simulink model "NewAuto_V1"  (R2021a)
settings: Solver=FixedStepAuto  StartTime=0.0  StopTime=inf  RelTol=1e-3
libraries: vexarmcortexlib x28, vexcommonlib x8
settings Model: ExtModeTrigDuration=25  Creator=nicoa  LastModifiedBy=Mihai Nicoara
settings SolverCC: AlgebraicLoopSolver=TrustRegion
settings OptimizationCC: EnhancedBackFolding=on  PassReuseOutputArgsAs=Individual arguments  ZeroExternalMemoryAtStartup=off  ZeroInternalMemoryAtStartup=off  MaxStackSize=64  OptimizeBlockOrder=speed  DifferentSizesBufferReuse=on  OptimizationCustomize=off  EfficientTunableParamExpr=on
settings DebuggingCC: ParameterTunabilityLossMsg=error  SFMachineParentedDataDiag=warning
settings HardwareCC: ProdBitPerPointer=32  ProdBitPerSizeT=32  ProdBitPerPtrDiffT=32  ProdLargestAtomicInteger=Long  ProdLargestAtomicFloat=Double  ProdWordSize=32  ProdHWDeviceType=ARM Compatible->ARM Cortex
settings SFSimCC: MATLABDynamicMemAlloc=off
settings RTWCC: SystemTargetFile=ert.tlc  HardwareBoard=ARM Cortex-based VEX Microcontroller  TLCOptions="-aInlineSetEventsForThisBaseRateFcn=TLC_FALSE -aSuppressMultiTaskScheduler=TLC_FALSE  -aRateBasedStepFcn=0"  TemplateMakefile=ert_default_tmf  GenerateReport=on  Toolchain=GNU Tools for VEX ARM Cortex  IncludeHyperlinkInReport=on  LaunchReport=on  GenerateTraceInfo=on  GenerateTraceReport=on  GenerateTraceReportSl=on  GenerateTraceReportSf=on  GenerateTraceReportEml=on
settings CodeAppCC: ForceParamTrailComments=on  IgnoreCustomStorageClasses=off  OperatorAnnotations=on  SimulinkDataObjDesc=on  SFDataObjDesc=on  InsertBlockDesc=on

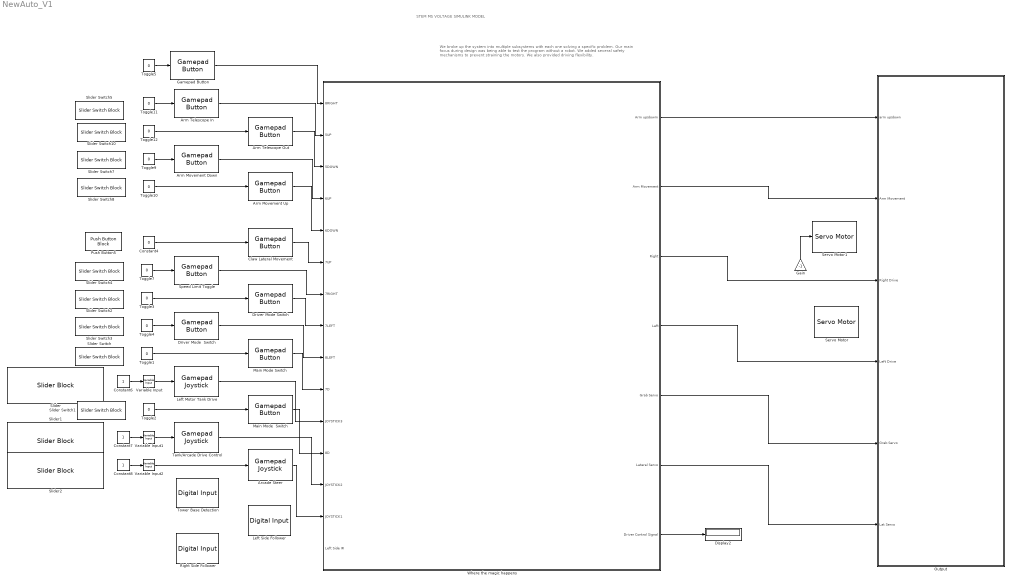
== system NewAuto_V1 ==
  note: We broke up the system into multiple subsystems with each one solving a specific problem. Our main focus during
      | design was being able to test the program without a robot. We added several safety mechanisms to prevent straining
      |  the motors. We also provided driving flexibility.
  note: STEM MS VOLTAGE SIMULINK MODEL
  "Arcade Steer " : vexarmcortexlib/Gamepad/Gamepad Joystick  joystick=1  chan=1  SimulationIn=on  SampleTime=0.02
      settings: SourceProductBaseCode=EC_VEX_MICRO
  Arm Movement Down : vexarmcortexlib/Gamepad/Gamepad Button  joystick=1  chan=6  button56=Down  button78=Down  SimulationIn=on  SampleTime=0.02
      settings: SourceProductBaseCode=EC_VEX_MICRO
  Arm Movement Up : vexarmcortexlib/Gamepad/Gamepad Button  joystick=1  chan=6  button56=Up  button78=Down  SimulationIn=on  SampleTime=0.02
      settings: SourceProductBaseCode=EC_VEX_MICRO
  Arm Telescope In : vexarmcortexlib/Gamepad/Gamepad Button  joystick=1  chan=5  button56=Down  button78=Down  SimulationIn=on  SampleTime=0.02
      settings: SourceProductBaseCode=EC_VEX_MICRO
  Arm Telescope Out : vexarmcortexlib/Gamepad/Gamepad Button  joystick=1  chan=5  button56=Up  button78=Down  SimulationIn=on  SampleTime=0.02
      settings: SourceProductBaseCode=EC_VEX_MICRO
  Claw Lateral Movement : vexarmcortexlib/Gamepad/Gamepad Button  joystick=1  chan=7  button56=Up  button78=Up  SimulationIn=on  SampleTime=0.02
      settings: SourceProductBaseCode=EC_VEX_MICRO
  Constant4 : Constant  Value=0
  Constant6 : Constant
  Constant7 : Constant
  Constant8 : Constant
  Display2 : Display
  Driver Mode  Switch : vexarmcortexlib/Gamepad/Gamepad Button  joystick=1  chan=8  button56=Up  button78=Left  SimulationIn=on  SampleTime=0.02
      settings: SourceProductBaseCode=EC_VEX_MICRO
  Driver Mode Switch : vexarmcortexlib/Gamepad/Gamepad Button  joystick=1  chan=7  button56=Up  button78=Left  SimulationIn=on  SampleTime=0.02
      settings: SourceProductBaseCode=EC_VEX_MICRO
  Gain : Gain  Gain=-1
  Gamepad Button : vexarmcortexlib/Gamepad/Gamepad Button  joystick=1  chan=8  button56=Up  button78=Right  SimulationIn=on  SampleTime=0.02
      settings: SourceProductBaseCode=EC_VEX_MICRO
  Left Motor Tank Drive : vexarmcortexlib/Gamepad/Gamepad Joystick  joystick=1  chan=3  SimulationIn=on  SampleTime=0.02
      settings: SourceProductBaseCode=EC_VEX_MICRO
  Left Side Follower : vexarmcortexlib/Sensors/Digital Input  inChan=1  SimulationIn=off  SampleTime=0.002
      settings: SourceProductBaseCode=EC_VEX_MICRO
  Main Mode  Switch : vexarmcortexlib/Gamepad/Gamepad Button  joystick=1  chan=8  button56=Up  button78=Down  SimulationIn=on  SampleTime=0.02
      settings: SourceProductBaseCode=EC_VEX_MICRO
  Main Mode Switch : vexarmcortexlib/Gamepad/Gamepad Button  joystick=1  chan=7  button56=Up  button78=Down  SimulationIn=on  SampleTime=0.02
      settings: SourceProductBaseCode=EC_VEX_MICRO
  Output : Subsystem
  Push Button5 : PushButtonBlock
  Right Side Follower : vexarmcortexlib/Sensors/Digital Input  inChan=6  SimulationIn=off  SampleTime=0.002
      settings: SourceProductBaseCode=EC_VEX_MICRO
  Servo Motor : vexarmcortexlib/Actuators/Servo Motor  motor=5  scaleFactor=60/127  SimulationOut=off
      settings: SourceProductBaseCode=EC_VEX_MICRO
  Servo Motor1 : vexarmcortexlib/Actuators/Servo Motor  motor=6  scaleFactor=60/127  SimulationOut=off
      settings: SourceProductBaseCode=EC_VEX_MICRO
  Slider : SliderBlock  LabelPosition=Hide  ScaleMin=-127  ScaleMax=127
  Slider Switch{,1..5,7..8,10} (9 alike) : SliderSwitchBlock  LabelPosition=Hide
      settings: Values={{'Off', 'On'}, [0 1]}
  Slider1 : SliderBlock  LabelPosition=Hide  ScaleMin=-127  ScaleMax=127
  Slider2 : SliderBlock  LabelPosition=Hide  ScaleMin=-127  ScaleMax=127
  Speed Limit Toggle : vexarmcortexlib/Gamepad/Gamepad Button  joystick=1  chan=7  button56=Up  button78=Right  SimulationIn=on  SampleTime=0.02
      settings: SourceProductBaseCode=EC_VEX_MICRO
  Tank/Arcade Drive Control : vexarmcortexlib/Gamepad/Gamepad Joystick  joystick=1  chan=2  SimulationIn=on  SampleTime=0.02
      settings: SourceProductBaseCode=EC_VEX_MICRO
  Toggle{1..5,7,9..12} (10 alike) : Constant  Value=0
      settings: OpenFcn=|
      | if strcmp('0',get_param(gcb, 'Value'))                        set_param(gcb, 'Value', '1');
      | else
      |             set_param(gcb, 'Value', '0');
      | end
  Tower Base Detection : vexarmcortexlib/Sensors/Digital Input  inChan=11  SimulationIn=off  SampleTime=0.002
      settings: SourceProductBaseCode=EC_VEX_MICRO
  Variable Input : vexarmcortexlib/Utilities/Variable Input  low=-127  gain=-29.69085144927537  high=127
      settings: SourceProductBaseCode=EC_VEX_MICRO
  Variable Input1 : vexarmcortexlib/Utilities/Variable Input  low=-127  gain=0  high=127
      settings: SourceProductBaseCode=EC_VEX_MICRO
  Variable Input2 : vexarmcortexlib/Utilities/Variable Input  low=-127  gain=0  high=127
      settings: SourceProductBaseCode=EC_VEX_MICRO
  Where the magic happens : Subsystem
  wires:
  Main Mode  Switch/1 -> Where the magic happens/12(8D)
  Main Mode Switch/1 -> Where the magic happens/10(7D)
  Driver Mode  Switch/1 -> Where the magic happens/9(8LEFT)
  Driver Mode Switch/1 -> Where the magic happens/8(7LEFT)
  Speed Limit Toggle/1 -> Where the magic happens/7(7RIGHT)
  Tank/Arcade Drive Control/1 -> Where the magic happens/13(JOYSTICK2)
  Left Motor Tank Drive/1 -> Where the magic happens/11(JOYSTICK3)
  "Arcade Steer "/1 -> Where the magic happens/14(JOYSTICK1)
  Claw Lateral Movement/1 -> Where the magic happens/6(7UP)
  Arm Movement Up/1 -> Where the magic happens/5(6DOWN)
  Arm Movement Down/1 -> Where the magic happens/4(6UP)
  Arm Telescope Out/1 -> Where the magic happens/3(5DOWN)
  Arm Telescope In/1 -> Where the magic happens/2(5UP)
  Toggle11/1 -> Arm Telescope In/1
  Toggle12/1 -> Arm Telescope Out/1
  Toggle9/1 -> Arm Movement Down/1
  Toggle10/1 -> Arm Movement Up/1
  Constant4/1 -> Claw Lateral Movement/1
  Toggle7/1 -> Speed Limit Toggle/1
  Toggle4/1 -> Driver Mode  Switch/1
  Toggle1/1 -> Main Mode Switch/1
  Constant6/1 -> Variable Input/1
  Variable Input/1 -> Left Motor Tank Drive/1
  Variable Input1/1 -> Tank/Arcade Drive Control/1
  Constant7/1 -> Variable Input1/1
  Variable Input2/1 -> "Arcade Steer "/1
  Constant8/1 -> Variable Input2/1
  Toggle2/1 -> Main Mode  Switch/1
  Toggle3/1 -> Driver Mode Switch/1
  Where the magic happens/7(Driver Control Signal) -> Display2/1
  Where the magic happens/6(Lateral Servo) -> Output/6(Lat Servo)
  Where the magic happens/5(Grab Servo) -> Output/5(Grab Servo)
  Where the magic happens/1(Arm up/dowm) -> Output/1(arm up/down)
  Where the magic happens/2(Arm Movement) -> Output/2(Arm Movement)
  Toggle5/1 -> Gamepad Button/1
  Gamepad Button/1 -> Where the magic happens/1(8RIGHT)
  Where the magic happens/3(Right) -> Output/3(Right Drive)
  Where the magic happens/4(Left) -> Output/4(Left Drive)
  ? -> Servo Motor/1, Gain/1
  Gain/1 -> Servo Motor1/1

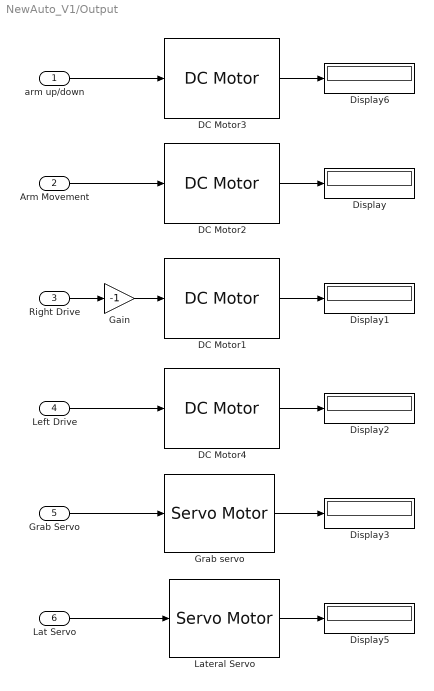
== system NewAuto_V1/Output ==
  arm up/down : Inport
  Arm Movement : Inport  Port=2
  Right Drive : Inport  Port=3
  Left Drive : Inport  Port=4
  Grab Servo : Inport  Port=5
  Lat Servo : Inport  Port=6
  DC Motor1 : vexarmcortexlib/Actuators/DC Motor  motor=2  scaleFactor=1/13.5  SimulationOut=on
      settings: SourceProductBaseCode=EC_VEX_MICRO
  DC Motor2 : vexarmcortexlib/Actuators/DC Motor  motor=4  scaleFactor=1/13.5  SimulationOut=on
      settings: SourceProductBaseCode=EC_VEX_MICRO
  DC Motor3 : vexarmcortexlib/Actuators/DC Motor  motor=7  scaleFactor=1/13.5  SimulationOut=on
      settings: SourceProductBaseCode=EC_VEX_MICRO
  DC Motor4 : vexarmcortexlib/Actuators/DC Motor  motor=9  scaleFactor=1/13.5  SimulationOut=on
      settings: SourceProductBaseCode=EC_VEX_MICRO
  Display{,1..3,5..6} (6 alike) : Display
  Gain : Gain  Gain=-1
  Grab servo : vexarmcortexlib/Actuators/Servo Motor  motor=3  scaleFactor=60/127  SimulationOut=on
      settings: SourceProductBaseCode=EC_VEX_MICRO
  Lateral Servo : vexarmcortexlib/Actuators/Servo Motor  motor=8  scaleFactor=60/127  SimulationOut=on
      settings: SourceProductBaseCode=EC_VEX_MICRO
  wires:
  Grab servo/1 -> Display3/1
  Arm Movement/1 -> DC Motor2/1
  Grab Servo/1 -> Grab servo/1
  DC Motor2/1 -> Display/1
  DC Motor3/1 -> Display6/1
  DC Motor4/1 -> Display2/1
  DC Motor1/1 -> Display1/1
  Lateral Servo/1 -> Display5/1
  arm up/down/1 -> DC Motor3/1
  Lat Servo/1 -> Lateral Servo/1
  Right Drive/1 -> Gain/1
  Left Drive/1 -> DC Motor4/1
  Gain/1 -> DC Motor1/1

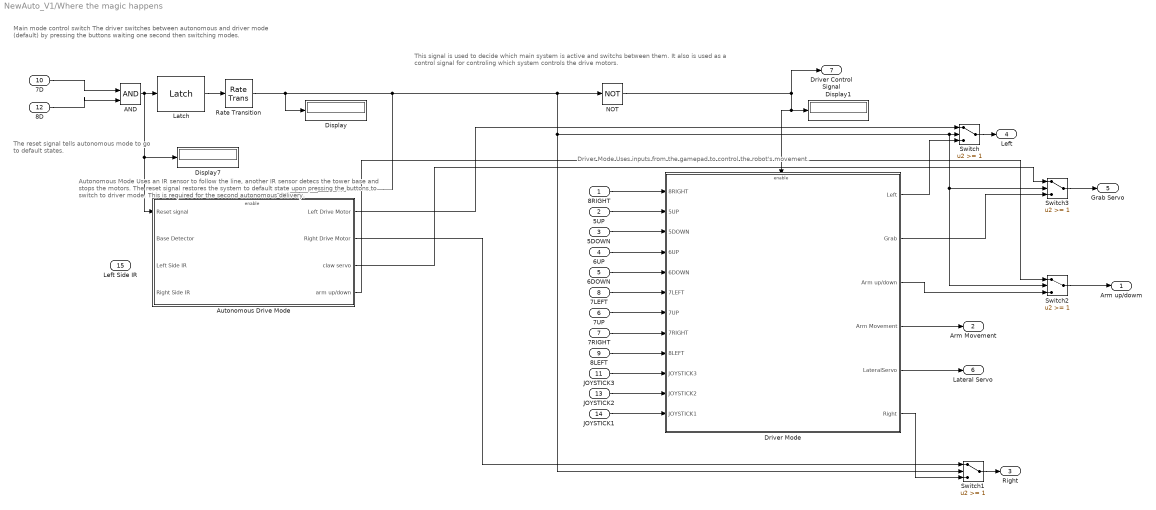
== system NewAuto_V1/Where the magic happens ==
  note: Driver Mode
      | Uses inputs from the gamepad to control the robot's movement.
  note: This signal is used to decide which main system is active and switchs between them.
      | It also is used as a control signal for controling which system controls the drive motors.
  note: The reset signal tells autonomous
      | mode to go to default states.
  note: Autonomous Mode
      | 	Uses an IR sensor to follow the line, another IR sensor detecs the
      | 	tower base and stops the motors. The reset signal restores the system
      | 	to default state upon pressing the buttons to switch to driver mode. This
      | 	is required for the second autonomous delivery.
  note: Main mode control switch
      | The driver switches between autonomous and driver mode (default) by
      | pressing the buttons waiting one second then switching modes.
  8RIGHT : Inport
  5UP : Inport  Port=2
  5DOWN : Inport  Port=3
  6UP : Inport  Port=4
  6DOWN : Inport  Port=5
  7UP : Inport  Port=6
  7RIGHT : Inport  Port=7
  7LEFT : Inport  Port=8
  8LEFT : Inport  Port=9
  7D : Inport  Port=10
  JOYSTICK3 : Inport  Port=11
  8D : Inport  Port=12
  JOYSTICK2 : Inport  Port=13
  JOYSTICK1 : Inport  Port=14
  Left Side IR : Inport  Port=15
  "AND " : Logic  IconShape=distinctive  AllPortsSameDT=off  OutDataTypeStr=boolean
  Autonomous Drive Mode : Subsystem
  Display : Display
  Display1 : Display
  Display7 : Display
  Driver Mode : Subsystem  TreatAsAtomicUnit=on
  Latch : vexcommonlib/Latch  output0=off  BlockPlatform=vexarmcortex
      settings: SourceProductBaseCode=EC_VEX_MICRO,VEXV5
  NOT : Logic  Operator=NOT  IconShape=distinctive  AllPortsSameDT=off  OutDataTypeStr=boolean
  Rate Transition : RateTransition
  Switch{,1..3} (4 alike) : Switch  Threshold=1
  Arm up/dowm : Outport
  Arm Movement : Outport  Port=2
  Right : Outport  Port=3
  Left : Outport  Port=4
  Grab Servo : Outport  Port=5
  Lateral Servo : Outport  Port=6
  Driver Control Signal : Outport  Port=7
  wires:
  7D/1 -> "AND "/1
  "AND "/1 -> Latch/1, Display7/1, Autonomous Drive Mode/1(Reset signal)
  8D/1 -> "AND "/2
  Rate Transition/1 -> Display/1, Autonomous Drive Mode/Enable, NOT/1, Switch1/2, Switch3/2, Switch2/2, Switch/2
  NOT/1 -> Display1/1, Driver Mode/Enable, Driver Control Signal/1
  Autonomous Drive Mode/1(Left Drive Motor) -> Switch/1
  Switch/1 -> Left/1
  Autonomous Drive Mode/2(Right Drive Motor) -> Switch1/1
  Switch1/1 -> Right/1
  7RIGHT/1 -> Driver Mode/8(7RIGHT)
  JOYSTICK3/1 -> Driver Mode/10(JOYSTICK3)
  JOYSTICK2/1 -> Driver Mode/11(JOYSTICK2)
  JOYSTICK1/1 -> Driver Mode/12(JOYSTICK1)
  7UP/1 -> Driver Mode/7(7UP)
  Driver Mode/4(Arm Movement) -> Arm Movement/1
  Driver Mode/1(Left) -> Switch/3
  5DOWN/1 -> Driver Mode/3(5DOWN)
  5UP/1 -> Driver Mode/2(5UP)
  6UP/1 -> Driver Mode/4(6UP)
  6DOWN/1 -> Driver Mode/5(6DOWN)
  7LEFT/1 -> Driver Mode/6(7LEFT)
  8LEFT/1 -> Driver Mode/9(8LEFT)
  Latch/1 -> Rate Transition/1
  Driver Mode/6(Right) -> Switch1/3
  Driver Mode/5(LateralServo) -> Lateral Servo/1
  8RIGHT/1 -> Driver Mode/1(8RIGHT)
  Switch2/1 -> Arm up/dowm/1
  Autonomous Drive Mode/4(arm up/down) -> Switch2/1
  Driver Mode/3(Arm up/down) -> Switch2/3
  Switch3/1 -> Grab Servo/1
  Autonomous Drive Mode/3(claw servo) -> Switch3/1
  Driver Mode/2(Grab) -> Switch3/3

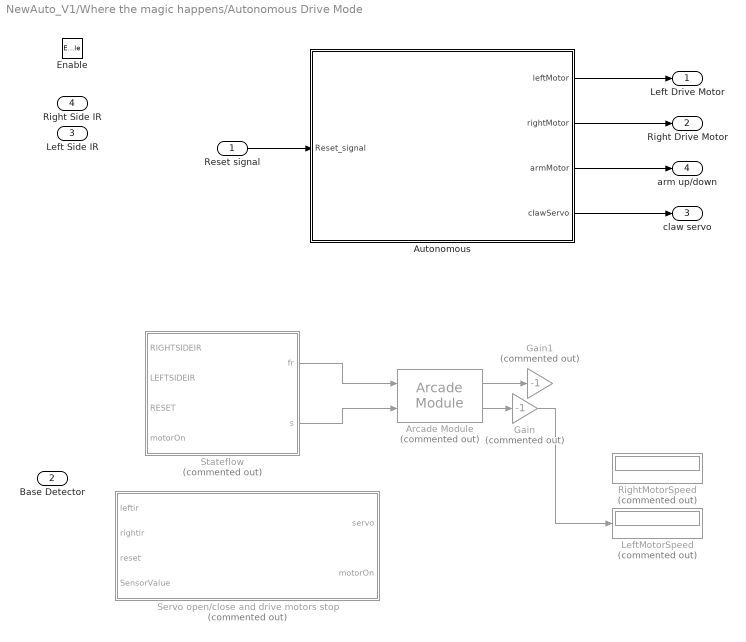
== system NewAuto_V1/Where the magic happens/Autonomous Drive Mode ==
  Reset signal : Inport
  Base Detector : Inport  Port=2
  Left Side IR : Inport  Port=3
  Right Side IR : Inport  Port=4
  Enable : EnablePort
  Arcade Module : vexcommonlib/Arcade Module  Commented=on  BlockPlatform=vexarmcortex
      settings: SourceProductBaseCode=EC_VEX_MICRO,VEXV5
  Autonomous : Stateflow chart  TreatAsAtomicUnit=on
  Gain : Gain  Commented=on  Gain=-1
  Gain1 : Gain  Commented=on  Gain=-1
  LeftMotorSpeed : Display  Commented=on
  RightMotorSpeed : Display  Commented=on
  Servo open/close and drive motors stop : Stateflow chart  Commented=on  TreatAsAtomicUnit=on
  Stateflow : Stateflow chart  Commented=on  TreatAsAtomicUnit=on
  Left Drive Motor : Outport
  Right Drive Motor : Outport  Port=2
  claw servo : Outport  Port=3
  arm up/down : Outport  Port=4
  wires:
  Stateflow/2(s) -> Arcade Module/2
  Stateflow/1(fr) -> Arcade Module/1
  Arcade Module/2 -> Gain/1
  Arcade Module/1 -> Gain1/1
  Gain/1 -> LeftMotorSpeed/1
  Autonomous/2(rightMotor) -> Right Drive Motor/1
  Autonomous/1(leftMotor) -> Left Drive Motor/1
  Autonomous/3(armMotor) -> arm up/down/1
  Autonomous/4(clawServo) -> claw servo/1
  Reset signal/1 -> Autonomous/1(Reset_signal)

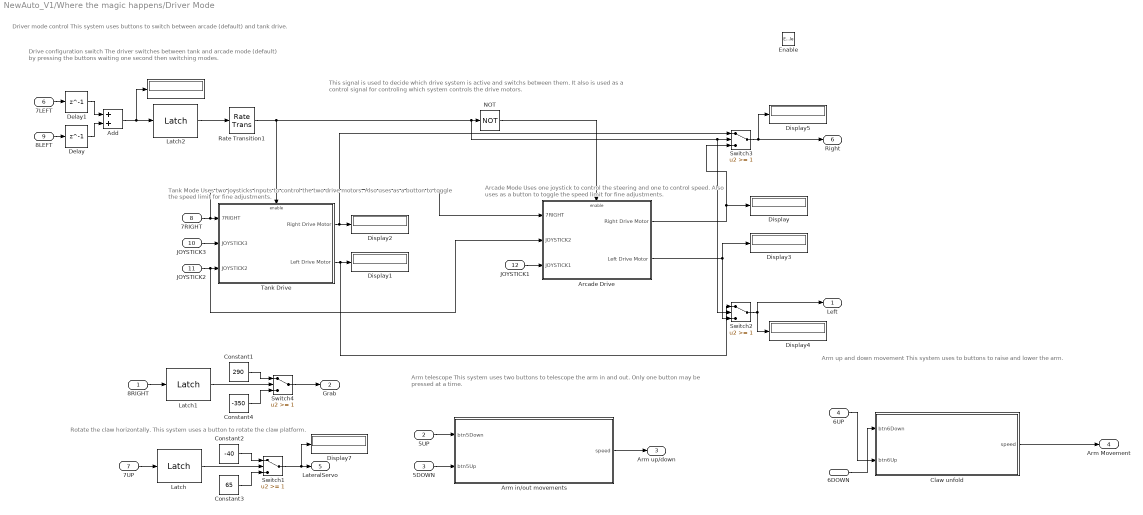
== system NewAuto_V1/Where the magic happens/Driver Mode ==
  note: Rotate the claw horizontally.
      | This system uses a button to rotate the claw platform.
  note: Arcade Mode
      | Uses one joystick to control the steering and one to control  speed.
      | Also uses as a button to toggle the speed limit for fine  adjustments.
  note: Tank Mode
      | Uses two joysticks inputs to control the two drive motors. Also uses as a button
      | to toggle the speed limit for fine adjustments.
  note: Drive configuration switch
      | The driver switches between tank and arcade mode (default) by
      | pressing the buttons waiting one second then switching modes.
  note: Arm telescope
      | This system uses two buttons to telescope the arm in and out.
      | Only one button may be pressed at a time.
  note: Arm up and down movement
      | This system uses to buttons to raise and lower the arm.
  note: Driver mode control
      | This system uses buttons to switch between arcade (default) and tank drive.
  note: This signal is used to decide which drive system is active and switchs between them.
      | It also is used as a control signal for controling which system controls the drive motors.
  8RIGHT : Inport
  5UP : Inport  Port=2
  5DOWN : Inport  Port=3
  6UP : Inport  Port=4
  6DOWN : Inport  Port=5
  7LEFT : Inport  Port=6
  7UP : Inport  Port=7
  7RIGHT : Inport  Port=8
  8LEFT : Inport  Port=9
  JOYSTICK3 : Inport  Port=10
  JOYSTICK2 : Inport  Port=11
  JOYSTICK1 : Inport  Port=12
  Enable : EnablePort
  " " : Display
  Add : Sum
  "Arcade Drive " : Subsystem  TreatAsAtomicUnit=on
  Arm in/out movements : Stateflow chart  TreatAsAtomicUnit=on
  Claw unfold : Stateflow chart  TreatAsAtomicUnit=on
  Constant1 : Constant  Value=290
  Constant2 : Constant  Value=-40
  Constant3 : Constant  Value=65
  Constant4 : Constant  Value=-350
  Delay : Delay  DelayLength=1  InitialCondition=0  SampleTime=0.5
  Delay1 : Delay  DelayLength=1  InitialCondition=0  SampleTime=0.5
  Display{,1..5,7} (7 alike) : Display
  Latch : vexcommonlib/Latch  output0=off  BlockPlatform=vexarmcortex
      settings: SourceProductBaseCode=EC_VEX_MICRO,VEXV5
  Latch1 : vexcommonlib/Latch  output0=off  BlockPlatform=vexarmcortex
      settings: SourceProductBaseCode=EC_VEX_MICRO,VEXV5
  Latch2 : vexcommonlib/Latch  output0=off  BlockPlatform=vexarmcortex
      settings: SourceProductBaseCode=EC_VEX_MICRO,VEXV5
  NOT : Logic  Operator=NOT  IconShape=distinctive  AllPortsSameDT=off  OutDataTypeStr=boolean
  Rate Transition1 : RateTransition  OutPortSampleTime=0.002
  Switch{1..4} (4 alike) : Switch  Threshold=1
  "Tank Drive " : Subsystem  TreatAsAtomicUnit=on
  Left : Outport
  Grab : Outport  Port=2
  Arm up/down : Outport  Port=3
  Arm Movement : Outport  Port=4
  LateralServo : Outport  Port=5
  Right : Outport  Port=6
  wires:
  Rate Transition1/1 -> NOT/1, Switch2/2, Switch3/2, "Tank Drive "/Enable
  7LEFT/1 -> Delay1/1
  NOT/1 -> "Arcade Drive "/Enable
  Delay1/1 -> Add/1
  Delay/1 -> Add/2
  Latch2/1 -> Rate Transition1/1
  Add/1 -> " "/1, Latch2/1
  8LEFT/1 -> Delay/1
  JOYSTICK3/1 -> "Tank Drive "/2(JOYSTICK3)
  JOYSTICK2/1 -> "Tank Drive "/3(JOYSTICK2), "Arcade Drive "/2(JOYSTICK2)
  JOYSTICK1/1 -> "Arcade Drive "/3(JOYSTICK1)
  7UP/1 -> Latch/1
  Latch/1 -> Switch1/2
  Switch1/1 -> Display7/1, LateralServo/1
  Constant2/1 -> Switch1/1
  Constant3/1 -> Switch1/3
  Switch2/1 -> Display4/1, Left/1
  "Arcade Drive "/2(Left Drive Motor) -> Switch2/3, Display3/1
  Switch3/1 -> Right/1, Display5/1
  "Arcade Drive "/1(Right Drive Motor) -> Display/1, Switch3/3
  7RIGHT/1 -> "Tank Drive "/1(7RIGHT), "Arcade Drive "/1(7RIGHT)
  "Tank Drive "/2(Left Drive Motor) -> Display1/1, Switch2/1
  "Tank Drive "/1(Right Drive Motor) -> Display2/1, Switch3/1
  6DOWN/1 -> Claw unfold/1(btn6Down)
  6UP/1 -> Claw unfold/2(btn6Up)
  Constant4/1 -> Switch4/3
  8RIGHT/1 -> Latch1/1
  Constant1/1 -> Switch4/1
  Latch1/1 -> Switch4/2
  Switch4/1 -> Grab/1
  Arm in/out movements/1(speed) -> Arm up/down/1
  5DOWN/1 -> Arm in/out movements/2(btn5Up)
  5UP/1 -> Arm in/out movements/1(btn5Down)
  Claw unfold/1(speed) -> Arm Movement/1

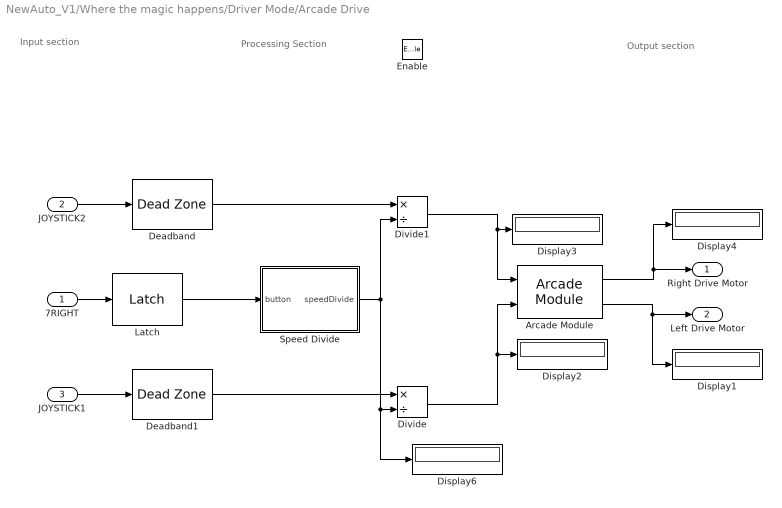
== system NewAuto_V1/Where the magic happens/Driver Mode/Arcade Drive  ==
  note: Output section
  note: Processing Section
  note: Input section
  7RIGHT : Inport
  JOYSTICK2 : Inport  Port=2
  JOYSTICK1 : Inport  Port=3
  Enable : EnablePort
  Arcade Module : vexcommonlib/Arcade Module  BlockPlatform=vexarmcortex
      settings: SourceProductBaseCode=EC_VEX_MICRO,VEXV5
  Deadband : DeadZone  LowerValue=-9  UpperValue=9  SaturateOnIntegerOverflow=on
  Deadband1 : DeadZone  LowerValue=-9  UpperValue=9  SaturateOnIntegerOverflow=on
  Display{1..4,6} (5 alike) : Display
  Divide : Product  Inputs=*/
  Divide1 : Product  Inputs=*/
  Latch : vexcommonlib/Latch  output0=off  BlockPlatform=vexarmcortex
      settings: SourceProductBaseCode=EC_VEX_MICRO,VEXV5
  Speed Divide : Stateflow chart  TreatAsAtomicUnit=on
  Right Drive Motor : Outport
  Left Drive Motor : Outport  Port=2
  wires:
  7RIGHT/1 -> Latch/1
  Speed Divide/1(speedDivide) -> Display6/1, Divide/2, Divide1/2
  Divide/1 -> Arcade Module/2, Display2/1
  Divide1/1 -> Arcade Module/1, Display3/1
  Arcade Module/1 -> Display4/1, Right Drive Motor/1
  Arcade Module/2 -> Display1/1, Left Drive Motor/1
  Latch/1 -> Speed Divide/1(button)
  JOYSTICK2/1 -> Deadband/1
  JOYSTICK1/1 -> Deadband1/1
  Deadband/1 -> Divide1/1
  Deadband1/1 -> Divide/1

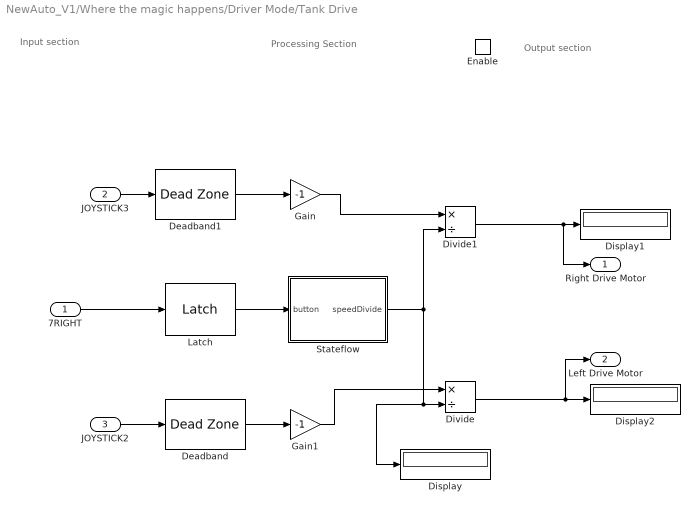
== system NewAuto_V1/Where the magic happens/Driver Mode/Tank Drive  ==
  note: Output section
  note: Processing Section
  note: Input section
  7RIGHT : Inport
  JOYSTICK3 : Inport  Port=2
  JOYSTICK2 : Inport  Port=3
  Enable : EnablePort
  Deadband : DeadZone  LowerValue=-9  UpperValue=9  SaturateOnIntegerOverflow=on
  Deadband1 : DeadZone  LowerValue=-9  UpperValue=9  SaturateOnIntegerOverflow=on
  Display : Display
  Display1 : Display
  Display2 : Display
  Divide : Product  Inputs=*/
  Divide1 : Product  Inputs=*/
  Gain : Gain  Gain=-1
  Gain1 : Gain  Gain=-1
  Latch : vexcommonlib/Latch  output0=off  BlockPlatform=vexarmcortex
      settings: SourceProductBaseCode=EC_VEX_MICRO,VEXV5
  Stateflow : Stateflow chart  TreatAsAtomicUnit=on
  Right Drive Motor : Outport
  Left Drive Motor : Outport  Port=2
  wires:
  7RIGHT/1 -> Latch/1
  Latch/1 -> Stateflow/1(button)
  Stateflow/1(speedDivide) -> Divide1/2, Display/1, Divide/2
  JOYSTICK3/1 -> Deadband1/1
  Divide1/1 -> Display1/1, Right Drive Motor/1
  Divide/1 -> Display2/1, Left Drive Motor/1
  JOYSTICK2/1 -> Deadband/1
  Gain/1 -> Divide1/1
  Gain1/1 -> Divide/1
  Deadband1/1 -> Gain/1
  Deadband/1 -> Gain1/1

== stateflow chart NewAuto_V1/Where the magic happens/Autonomous Drive Mode/Servo open//close and drive motors stop ==
  state move
    entry:
    servo = 0;
    motorOn = 1;
  state PreStop
    entry:
    servo = 0;
    motorOn = 1;
  state off
    entry:
    servo = 0;
    motorOn = 0;
  state PreOff
    entry:
    servo= -110;
    motorOn = 2;
  state Stop
    entry:
    servo = 110;
    motorOn = 0;
  (default) -> move
  move -> PreStop : [SensorValue == 1 && leftir == 1 && rightir == 1 && motorOn == 1]
  off -> move : [reset == 0 && SensorValue == 1 && leftir == 1 && rightir == 1]
  PreStop -> Stop [order 2] : [after(1,sec)]
  PreStop -> move [order 1] : [rightir == 0 || leftir == 0 || SensorValue == 0]
  PreOff -> off : [after(1,sec)]
  Stop -> PreOff : [after(1,sec)]
  data: leftir input; rightir input; reset input; SensorValue input; servo output; motorOn output

== stateflow chart NewAuto_V1/Where the magic happens/Driver Mode/Arm in//out movements ==
  state ARMDOWN
    entry:
    speed = -100;
  state STOPPED
    entry:
    speed = 0;
  state ARMUP
    entry:
    speed = 80;
  (default) -> STOPPED
  STOPPED -> ARMUP [order 1] : [btn5Down == 0 && btn5Up == 1 ]
  STOPPED -> ARMDOWN [order 2] : [btn5Down == 1 && btn5Up == 0]
  ARMDOWN -> STOPPED [order 2] : [btn5Down == 0]
  ARMUP -> STOPPED [order 2] : [btn5Up == 0]
  ARMDOWN -> STOPPED [order 1] : [btn5Down == 1 && btn5Up == 1]
  ARMUP -> STOPPED [order 1] : [btn5Down == 1 && btn5Up == 1]
  data: btn5Down input; btn5Up input; speed output

== stateflow chart NewAuto_V1/Where the magic happens/Driver Mode/Claw unfold ==
  state ARMDOWN
    entry:
    speed = -50;
  state STOPPED
    entry:
    speed = 0;
  state ARMUP
    entry:
    speed = 140;
  (default) -> STOPPED
  STOPPED -> ARMUP [order 1] : [btn6Down == 0 && btn6Up == 1 ]
  STOPPED -> ARMDOWN [order 2] : [btn6Down == 1 && btn6Up == 0]
  ARMDOWN -> STOPPED [order 2] : [btn6Down == 0]
  ARMUP -> STOPPED [order 2] : [btn6Up == 0]
  ARMDOWN -> STOPPED [order 1] : [btn6Down == 1 && btn6Up == 1]
  ARMUP -> STOPPED [order 1] : [btn6Down == 1 && btn6Up == 1]
  data: speed output; btn6Down input; btn6Up input

== stateflow chart NewAuto_V1/Where the magic happens/Autonomous Drive Mode/Autonomous ==
  state Start
    entry:
    leftMotor = 0;
    rightMotor = 0;
    armMotor = 0;
    clawServo = 350;
  state A
    entry:
    leftMotor = 0;
    rightMotor = 0;
    armMotor = -40;
    clawServo = 200;
  state B
    entry:
    leftMotor = -100;
    rightMotor = -100;
    armMotor = 0;
  state E
    entry:
    leftMotor = 0;
    rightMotor = 0;
    armMotor = 40;
  state C
    entry:
    leftMotor = 0;
    rightMotor = 0;
    armMotor = 0;
  state D
    entry:
    leftMotor = 100;
    rightMotor = 100;
    armMotor = 0;
  state F
    entry:
    leftMotor = 0;
    rightMotor = 0;
    armMotor =  0;
    clawServo = -200;
  state G
    entry:
    leftMotor = 0;
    rightMotor = 0;
    armMotor =  -40;
    clawServo = -200;
  state H
    entry:
    leftMotor = -100;
    rightMotor = -100;
    armMotor =  -40;
    clawServo = -200;
  state I
    entry:
    leftMotor = 0;
    rightMotor = 0;
    armMotor =  0;
    clawServo = -200;
  (default) -> Start
  Start -> A : [after(1,sec)]
  A -> B : [after(1,sec)]
  I -> Start : [after(5,sec)]
  B -> C : [after(1, sec)]
  C -> D : [after(1,sec)]
  D -> E : [after(0.92,sec)]
  E -> F : [after(1,sec)]
  F -> G : [after(1,sec)]
  G -> H : [after(2.5,sec)]
  H -> I : [after(1,sec)]
  data: leftMotor output; rightMotor output; armMotor output; clawServo output; Reset_signal input

== stateflow chart NewAuto_V1/Where the magic happens/Autonomous Drive Mode/Stateflow ==
  state STRAIGHT
    entry:
    fr = 110;
    s = 0;
  state GO_RIGHT
    entry:
    fr = 90;
    s = -110;
  state GO_LEFT
    entry:
    fr = 90;
    s = 110;
  state BackUp
    entry:
    fr = -30;
    s = 30;
  state STOP
    entry:
    fr = 0;
    s = 0;
  (default) -> STRAIGHT
  GO_LEFT -> STRAIGHT [order 3] : [LEFTSIDEIR == 0 && RIGHTSIDEIR == 0]
  GO_RIGHT -> STRAIGHT [order 3] : [RIGHTSIDEIR == 0 && LEFTSIDEIR == 0]
  STRAIGHT -> GO_RIGHT [order 3] : [RIGHTSIDEIR == 0 && LEFTSIDEIR == 1]
  STRAIGHT -> GO_LEFT [order 2] : [LEFTSIDEIR == 0 && RIGHTSIDEIR ==1]
  STOP -> STRAIGHT [order 3] : [RIGHTSIDEIR == 0 && LEFTSIDEIR == 0 && RESET == 0]
  STRAIGHT -> STOP [order 1] : [motorOn == 0]
  GO_LEFT -> GO_RIGHT [order 2] : [LEFTSIDEIR == 1 && RIGHTSIDEIR == 0]
  GO_RIGHT -> GO_LEFT [order 2] : [RIGHTSIDEIR == 1 && LEFTSIDEIR == 0]
  STOP -> GO_LEFT [order 2] : [RESET == 0 && LEFTSIDEIR == 0]
  GO_LEFT -> STOP [order 1] : [motorOn == 0]
  STOP -> GO_RIGHT [order 1] : [RESET == 0 && RIGHTSIDEIR == 0]
  GO_RIGHT -> STOP [order 1] : [motorOn == 0]
  BackUp -> STOP : [motorOn == 2]
  STOP -> BackUp [order 4] : [motorOn ==2]
  data: RIGHTSIDEIR input; LEFTSIDEIR input; RESET input; motorOn input; fr output; s output

== stateflow chart NewAuto_V1/Where the magic happens/Driver Mode/Arcade Drive /Speed Divide ==
  state Full_Speed
    entry:
    speedDivide = 1
  state Slow_Speed
    entry:
    speedDivide = 2
  (default) -> Full_Speed
  Full_Speed -> Slow_Speed : [button == 1]
  Slow_Speed -> Full_Speed : [button == 0]
  data: speedDivide output; button input

== stateflow chart NewAuto_V1/Where the magic happens/Driver Mode/Tank Drive /Stateflow ==
  state Full_Speed
    entry:
    speedDivide = 1
  state Slow_Speed
    entry:
    speedDivide = 2
  (default) -> Full_Speed
  Full_Speed -> Slow_Speed : [button]
  Slow_Speed -> Full_Speed : [button == 0]
  data: speedDivide output; button input
